simulink model "split_junction_test"  (R2014b)
settings: Solver=ode23tb  StartTime=0.0  StopTime=200  RelTol=1e-3
libraries: DAEMOT_Lib x8
settings Model: Creator=pangbor2  LastModifiedBy=koeln2

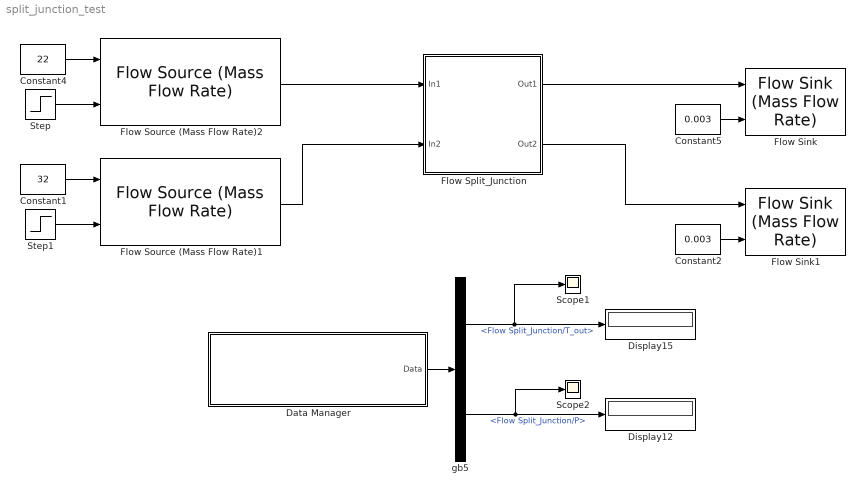
== system split_junction_test ==
  Constant1 : Constant  Value=32
  Constant2 : Constant  Value=0.003
  Constant4 : Constant  Value=22
  Constant5 : Constant  Value=0.003
  Data Manager : Subsystem  AncestorBlock=DAEMOT_Lib/Support Functions/Data Manager  mask{null=0}
      mask init:
      | set_param(gcb, 'LinkStatus', 'inactive')    % disable the library link
      settings: OpenFcn=data_manager
      mask Display: str ='Flow Split_Junction/T_out\nFlow Split_Junction/P'; fprintf(str)
  Display12 : Display
  Display15 : Display
  Flow Sink : DAEMOT_Lib/Components/Flow Sink (Mass Flow Rate)  M_ext=on  M=0  T_ext=on  T=0  P_ext=on  P=0
  Flow Sink1 : DAEMOT_Lib/Components/Flow Sink (Mass Flow Rate)  M_ext=on  M=0  T_ext=on  T=0  P_ext=on  P=0
  Flow Source (Mass Flow Rate)1 : DAEMOT_Lib/Components/Flow Source (Mass Flow Rate)  M_ext=on  M=0  T_ext=on  T=0  P_ext=on  P=0
  Flow Source (Mass Flow Rate)2 : DAEMOT_Lib/Components/Flow Source (Mass Flow Rate)  M_ext=on  M=0  T_ext=on  T=0  P_ext=on  P=0
  Flow Split_Junction : Subsystem  AncestorBlock=DAEMOT_Lib/Components/Flow Split_Junction  mask(Split/Junction){fld=PG50, Num_Out=2, Num_In=2, P_init=110, T_init=22, D=0.013, L=0.1, t=0.0015, E=2.4e6, v=0.4}
      mask prompts: fld "Fluid Type"; Num_Out "Number of Outlet Flows"; Num_In "Number of Inlet Flows"; P_init "Initial Pressure [kPa]"; T_init "Initial Temperature [°C]"; D "Diameter [m]"; L "Length [m]"; t "Tube Wall Thickness [m]"; E "Tube Modulus of Elasticity [kPa]"; v "Tube Poisson Ratio [-]"
      mask help: Splits and junctions flows using dynamic relationships. Note that the library link of the block is disabled when it is imported into a model.
      mask init:
      | h      = get_param(gcb,'handle');   % Get block handle
      | blk    = gcb;
      | hblock = get(h);     % Parse out handles structure
      | 
      | load('Fluids.mat');
      | Fluid = eval(['Fluid.',fld]);
      | 
      | % delete any previous inports and bus selectors
      | for i = str2num(hblock.Num_In)+1:hblock.Ports(1)
      |     delete_block([blk,'/In',num2str(i)])
      |     delete_block([blk,'/gb',num2str(i)])
      |     delete_block([blk,'/gm',num2str(i)])
      |     delete_block([blk,'/gt',num2str(i)])
      |     delete_block([blk,'/gp',num2str(i)])
      |     delete_block([blk,'/Sink',num2str(i)])
      |     delete_block([blk,'/pout',num2str(i)])
      |     delete_block([blk,'/min',num2str(i)])
      |     delete_block([blk,'/tin',num2str(i)])
      |     
      |     delete_unconnected_lines(blk)
      | end
      | 
      | % delete any previous inports and bus selectors
      | for i = str2num(hblock.Num_Out)+1:hblock.Ports(2)
      |     delete_block([blk,'/Out',num2str(i)])
      |     delete_block([blk,'/m',num2str(i)])
      |     delete_block([blk,'/t',num2str(i)])
      |     delete_block([blk,'/p',num2str(i)])
      |     delete_block([blk,'/b',num2str(i)])
      |     delete_block([blk,'/Source',num2str(i)])
      |     delete_block([blk,'/g',num2str(i)])
      |     delete_block([blk,'/mout',num2str(i)])
      |     %delete_block([blk,'/tout',num2str(i)])
      |     
      |     delete_unconnected_lines(blk)
      | end
      | 
      | set_param([blk,'/Mux_In_1'],'Inputs',hblock.Num_In)
      | set_param([blk,'/Mux_In_2'],'Inputs',hblock.Num_Out)
      | set_param([blk,'/Mux_In_3'],'Inputs',hblock.Num_In)
      | %set_param([blk,'/Mux_Out_1'],'Outputs',hblock.Num_Out)
      | 
      | % generate inports, bus selectors, and route lines to each vector concat
      | for i = hblock.Ports(1)+1:str2num(hblock.Num_In)
      |     
      |     % add blocks
      |     add_block('simulink/Ports & Subsystems/In1',   [blk,'/In',num2str(i)],    'Position',[120 i*80-25+20 150 i*80-12+20]);         % adding inport
      |     add_block([blk,'/gb1'],                        [blk,'/gb',num2str(i)],   'Position',[200 i*80-20+20-18 205 i*80-2+20+2]);         % adding inport
      |     add_block('simulink/Signal Routing/Goto',      [blk,'/gm',num2str(i)],    'Position',[260 i*80-17 340 i*80-3]);         % adding inport
      |     add_block('simulink/Signal Routing/Goto',      [blk,'/gt',num2str(i)],    'Position',[260 i*80+3 340 i*80+17]);         % adding inport
      |     add_block('simulink/Sinks/Terminator',          [blk,'/gp',num2str(i)],    'Position',[260 i*80+23 280 i*80+37]);         % adding inport
      |     add_block('DAEMOT_Lib/Support Functions/Sink',[blk,'/Sink',num2str(i)],'Position',[745 i*80-14 810 i*80+14]);         % adding inport
      |     add_block('simulink/Signal Routing/From',      [blk,'/pout',num2str(i)],    'Position',[625 i*80-14 705 i*80+14]);         % adding inport
      |     add_block('simulink/Signal Routing/From',       [blk,'/min',num2str(i)],     'Position',[935 -258+i*20 1015 -242+i*20]);         % adding inport
      |     add_block('simulink/Signal Routing/From',       [blk,'/tin',num2str(i)],     'Position',[935 1+i*20 1015 19+i*20]);         % adding inport
      |     
      |     % set goto and from tags
      |     set_param([blk,'/gm',num2str(i)],'GotoTag',char(horzcat('M_in',num2str(i))))
      |     set_param([blk,'/gt',num2str(i)],'GotoTag',char(horzcat('T_in',num2str(i))))
      |     %set_param([blk,'/gp',num2str(i)],'GotoTag',char(horzcat('P_in',num2str(i))))
      |     set_param([blk,'/pout',num2str(i)],'GotoTag',char('P'))
      |     set_param([blk,'/min',num2str(i)],'GotoTag',char(horzcat('M_in',num2str(i))))
      |     set_param([blk,'/tin',num2str(i)],'GotoTag',char(horzcat('T_in',num2str(i))))
      |     
      |     % set goto and from background colors
      |     set_param([blk,'/gm',num2str(i)],'BackgroundColor','yellow')
      |     set_param([blk,'/gt',num2str(i)],'BackgroundColor','yellow')
      |     %set_param([blk,'/gp',num2str(i)],'BackgroundColor','yellow')
      |     set_param([blk,'/min',num2str(i)],'BackgroundColor','yellow')
      |     set_param([blk,'/tin',num2str(i)],'BackgroundColor','yellow')
      |     set_param([blk,'/pout',num2str(i)],'BackgroundColor','cyan')
      |     
      |     % add lines
      |     add_line(blk,['In',num2str(i),'/1'], ['gb',num2str(i),'/1'],'AutoRouting','on')
      |     add_line(blk,['gb',num2str(i),'/1'],  ['gm',num2str(i),'/1'],'AutoRouting','on')
      |     add_line(blk,['gb',num2str(i),'/2'],  ['gt',num2str(i),'/1'],'AutoRouting','on')
      |     add_line(blk,['gb',num2str(i),'/3'],  ['gp',num2str(i),'/1'],'AutoRouting','on')
      |     add_line(blk,['pout',num2str(i),'/1'],  ['Sink',num2str(i),'/1'],'AutoRouting','on')
      |     add_line(blk,['min',num2str(i),'/1'],  ['Mux_In_1/',num2str(i)],'AutoRouting','on')
      |     add_line(blk,['tin',num2str(i),'/1'],  ['Mux_In_3/',num2str(i)],'AutoRouting','on')
      |     
      | end
      | 
      | % generate inports, bus selectors, and route lines to each vector concat
      | for i = hblock.Ports(2)+1:str2num(hblock.Num_Out)
      |     
      |     % add blocks
      |     add_block('simulink/Ports & Subsystems/Out1',   [blk,'/Out',num2str(i)],   'Position',[30 i*80-25+20 60 i*80-12+20]);         % adding inport
      |     add_block('simulink/Signal Routing/From',       [blk,'/m',num2str(i)],     'Position',[-150 i*80-20 -70 i*80-2]);         % adding inport
      |     add_block('simulink/Signal Routing/From',       [blk,'/t',num2str(i)],     'Position',[-150 i*80-20+20 -70 i*80-2+20]);         % adding inport
      |     add_block('simulink/Signal Routing/From',       [blk,'/p',num2str(i)],     'Position',[-150 i*80-20+40 -70 i*80-2+40]);         % adding inport
      |     add_block('simulink/Signal Routing/Bus Creator',[blk,'/b',num2str(i)],     'Position',[5 i*80-20+20-18 10 i*80-2+20+2]);         % adding inport
      |     add_block('DAEMOT_Lib/Support Functions/Source',[blk,'/Source',num2str(i)],'Position',[395 i*80-14 460 i*80+14]);         % adding inport
      |     add_block('simulink/Signal Routing/Goto',       [blk,'/g',num2str(i)],     'Position',[505 i*80-9 585 i*80+9]);         % adding inport
      |     add_block('simulink/Signal Routing/From',       [blk,'/mout',num2str(i)],  'Position',[935 -129+i*20 1015 -111+i*20]);         % adding inport
      |     %add_block('simulink/Signal Routing/Goto',      [blk,'/tout',num2str(i)],   'Position',[1455 -259+i*20 1535 -241+i*20]);         % adding inport
      |     
      |     % set goto and from tags
      |     set_param([blk,'/m',num2str(i)],'GotoTag',char(horzcat('M_out',num2str(i))))
      |     %set_param([blk,'/t',num2str(i)],'GotoTag',char(horzcat('T_out',num2str(i))))
      |     set_param([blk,'/t',num2str(i)],'GotoTag',char('T'))
      |     set_param([blk,'/p',num2str(i)],'GotoTag',char('P'))
      |     set_param([blk,'/g',num2str(i)],'GotoTag',char(horzcat('M_out',num2str(i))))
      |     set_param([blk,'/mout',num2str(i)],'GotoTag',char(horzcat('M_out',num2str(i))))
      |     %set_param([blk,'/tout',num2str(i)],'GotoTag',char(horzcat('T_out',num2str(i))))
      |     set_param([blk,'/b',num2str(i)],'Inputs','3')
      |     
      |     % set goto and from background colors
      |     set_param([blk,'/t',num2str(i)],'BackgroundColor','cyan')
      |     set_param([blk,'/m',num2str(i)],'BackgroundColor','cyan')
      |     set_param([blk,'/p',num2str(i)],'BackgroundColor','cyan')
      |     set_param([blk,'/g',num2str(i)],'BackgroundColor','cyan')
      |     set_param([blk,'/mout',num2str(i)],'BackgroundColor','cyan')
      |     %set_param([blk,'/tout',num2str(i)],'BackgroundColor','cyan')
      |     
      |     % add lines
      |     add_line(blk,['m',num2str(i),'/1'],['b',num2str(i),'/1'],'AutoRouting','on')
      |     p = get_param([blk,'/m',num2str(i)],'PortHandles');
      |     l = get_param(p.Outport,'Line');
      |     set_param(l,'Name','mdot_kgps')
      |     
      |     add_line(blk,['t',num2str(i),'/1'],['b',num2str(i),'/2'],'AutoRouting','on')
      |     p = get_param([blk,'/t',num2str(i)],'PortHandles');
      |     l = get_param(p.Outport,'Line');
      |     set_param(l,'Name','T_C')
      |     
      |     add_line(blk,['p',num2str(i),'/1'],['b',num2str(i),'/3'],'AutoRouting','on')
      |     p = get_param([blk,'/p',num2str(i)],'PortHandles');
      |     l = get_param(p.Outport,'Line');
      |     set_param(l,'Name','P_kPa')
      |     
      |     add_line(blk,['b',num2str(i),'/1'],['Out',num2str(i),'/1'],'AutoRouting','on')
      |     add_line(blk,['Source',num2str(i),'/1'],['g',num2str(i),'/1'],'AutoRouting','on')
      |     add_line(blk,['mout',num2str(i),'/1'],  ['Mux_In_2/',num2str(i)],'AutoRouting','on')
      |     %add_line(blk,['Mux_Out_1/',num2str(i)], ['tout',num2str(i),'/1'],'AutoRouting','on')
      | end
      | 
      | try
      |     set_param([blk,'/Selector1'],'InputPortWidth',num2str(hblock.Num_In))
      |     
      |     selector_str = '[1 ';
      |     for i = 2:str2num(hblock.Num_In)
      |         selector_str = [selector_str,num2str(i),' '];
      |     end
      |     selector_str = [selector_str,']'];
      |     set_param([blk,'/Selector1'],'IndexParamArray',{selector_str})%num2cell(1:hblock.Num_In))
      | catch
      |     selector_str = '[1 ';
      |     for i = 2:str2num(hblock.Num_In)
      |         selector_str = [selector_str,num2str(i),' '];
      |     end
      |     selector_str = [selector_str,']'];
      |     set_param([blk,'/Selector1'],'IndexParamArray',{selector_str})%num2cell(1:hblock.Num_In))
      |     
      |     set_param([blk,'/Selector1'],'InputPortWidth',num2str(hblock.Num_In))
      | end 
      |     
      |     clear h blk hblock
      settings: CopyFcn=|
      | h      = get_param(gcb,'handle');   % Get block handle
      | blk    = gcb;
      | 
      | set_param(blk, 'LinkStatus', 'inactive')
      settings: OpenFcn=|
      | load('Fluids.mat');
      | Set_Fluid_Popup_Names( Fluid )
      mask TypeOptions fld: Fuel | Water | Air | PG50
      mask DialogControl Container15 Prompt: Component Sizing - Nominal Values
      mask Display:
      | image(imread('Split.jpg'));
      | 
      | text(0.5,0.95,['{\bf',fld,' Split/Junction}'],'TexMode','on','horizontalAlignment', 'center')
      | text(0.5,0.08,['{(P)}'],'TexMode','on','horizontalAlignment', 'center')
      | 
      | h      = get_param(gcb,'handle');   % Get block handle
      | blk    = gcb;
      | hblock = get(h);     % Parse out handles structure
      | for i = 1:str2num(hblock.Num_In)
      |     port_label('input',i,horzcat('Flow In #',num2str(i)))
      | end
      | for i = 1:str2num(hblock.Num_Out)
      |     port_label('output',i,horzcat('Flow Out #',num2str(i)))
      | end
  Scope1 : Scope
  Scope2 : Scope
  Step : Step  Time=100  Before=.002  After=.003  SampleTime=0
  Step1 : Step  Time=100  Before=.004  After=.003  SampleTime=0
  gb5 : BusSelector  OutputSignals=Flow Split_Junction/T_out,Flow Split_Junction/P
  wires:
  Constant5/1 -> Flow Sink/2
  Flow Split_Junction/1(Out1) -> Flow Sink/1
  Flow Source (Mass Flow Rate)2/1 -> Flow Split_Junction/1(In1)
  Constant2/1 -> Flow Sink1/2
  Flow Split_Junction/2(Out2) -> Flow Sink1/1
  Flow Source (Mass Flow Rate)1/1 -> Flow Split_Junction/2(In2)
  Data Manager/1(Data) -> gb5/1
  gb5/2 -> Display12/1, Scope2/1  "<Flow Split_Junction/P>"
  gb5/1 -> Display15/1, Scope1/1  "<Flow Split_Junction/T_out>"
  Constant4/1 -> Flow Source (Mass Flow Rate)2/1
  Constant1/1 -> Flow Source (Mass Flow Rate)1/1
  Step/1 -> Flow Source (Mass Flow Rate)2/2
  Step1/1 -> Flow Source (Mass Flow Rate)1/2

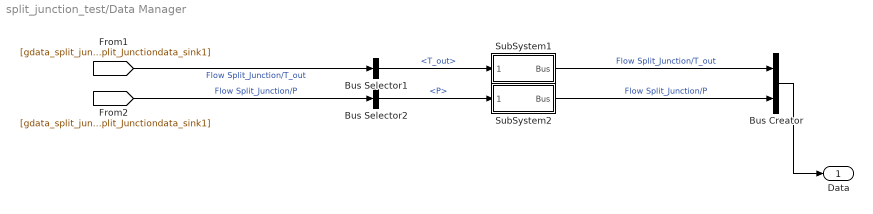
== system split_junction_test/Data Manager ==
  Bus Creator : BusCreator  Inputs=2
  Bus Selector1 : BusSelector  OutputSignals=T_out
  Bus Selector2 : BusSelector  OutputSignals=P
  SubSystem1 : Subsystem
  SubSystem2 : Subsystem
  Data : Outport
  wires:
  Bus Creator/1 -> Data/1
  [gdata_split_junction_testFlowSplit_Junctiondata_sink1] -> Bus Selector1/1  "Flow Split_Junction/T_out"
  Bus Selector1/1 -> SubSystem1/1(Rename)  "<T_out>"
  SubSystem1/1(Bus) -> Bus Creator/1  "Flow Split_Junction/T_out"
  [gdata_split_junction_testFlowSplit_Junctiondata_sink1] -> Bus Selector2/1  "Flow Split_Junction/P"
  Bus Selector2/1 -> SubSystem2/1(Rename)  "<P>"
  SubSystem2/1(Bus) -> Bus Creator/2  "Flow Split_Junction/P"

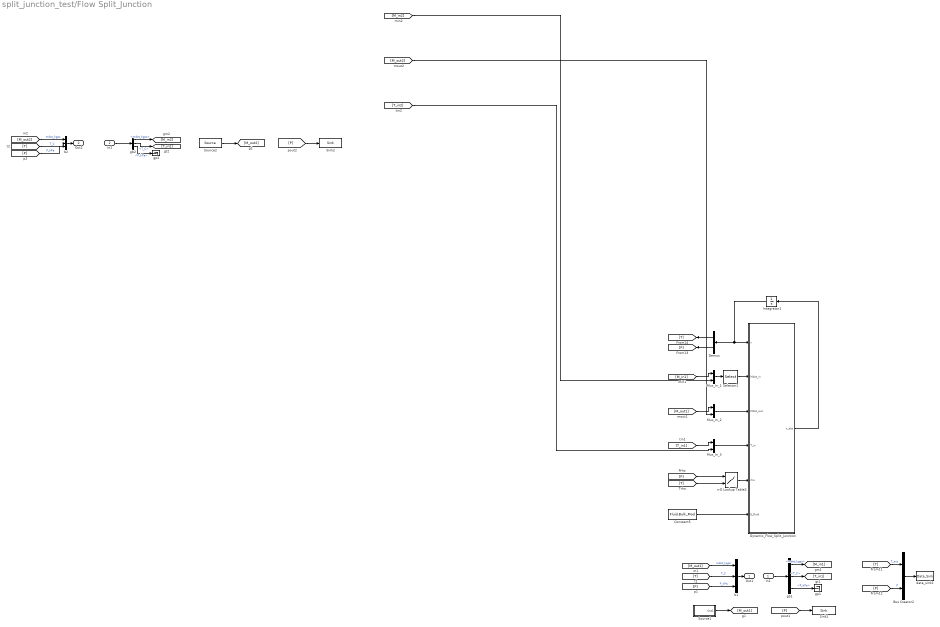
== system split_junction_test/Flow Split_Junction ==
  In1 : Inport
  In2 : Inport  Port=2
  Bus Creator2 : BusCreator  Inputs=2
  Constant5 : Constant  Value=Fluid.Bulk_Mod
  Demux : Demux  Outputs=2
  Dynamic_Flow_Split_Junction : MATLAB Function  TreatAsAtomicUnit=on
  Integrator1 : Integrator  InitialCondition=[T_init P_init]
  Mux_In_1 : Mux  Inputs=2
  Mux_In_2 : Mux  Inputs=2
  Mux_In_3 : Mux  Inputs=2
  Selector1 : Selector  InputPortWidth=2  Indices=[1 2 ]
  Sink1 : DAEMOT_Lib/Support Functions/Sink
  Sink2 : DAEMOT_Lib/Support Functions/Sink
  Source1 : Subsystem
      mask init:
      | n_src = gcb;
      | n_src = str2num(n_src(end));
      | 
      | rev_comms_source(n_src);
      mask Display: text(0.25,0.5,'Source')
  Source2 : DAEMOT_Lib/Support Functions/Source
  b1 : BusCreator  Inputs=3
  b2 : BusCreator  Inputs=3
  data_sink1 : DAEMOT_Lib/Support Functions/Data_Sink
  gb1 : BusSelector  OutputSignals=mdot_kgps,T_C,P_kPa
  gb2 : BusSelector  OutputSignals=mdot_kgps,T_C,P_kPa
  gp1 : Terminator
  gp2 : Terminator
  n-D Lookup Table2 : Lookup_n-D  BreakpointsForDimension1=Fluid.P  BreakpointsForDimension2=Fluid.T  BreakpointsForDimension3=[5, 7]  Table=Fluid.Rho_pt  ExtrapMethod=Clip  UseLastTableValue=on  RndMeth=Simplest  InputSameDT=on
  Out1 : Outport
  Out2 : Outport  Port=2
  wires:
  b1/1 -> Out1/1
  [M_out1] -> b1/1  "mdot_kgps"
  gb1/2 -> [T_in1]  "<T_C>"
  [T] -> b1/2  "T_C"
  gb1/1 -> [M_in1]  "<mdot_kgps>"
  Source1/1(Out1) -> [M_out1]
  In1/1 -> gb1/1
  [P] -> b1/3  "P_kPa"
  gb1/3 -> gp1/1  "<P_kPa>"
  Mux_In_3/1 -> Dynamic_Flow_Split_Junction/4(T_in)
  Mux_In_1/1 -> Selector1/1
  Mux_In_2/1 -> Dynamic_Flow_Split_Junction/3(Mdot_out)
  [M_in1] -> Mux_In_1/1
  [M_out1] -> Mux_In_2/1
  [T_in1] -> Mux_In_3/1
  [P] -> Sink1/1
  Dynamic_Flow_Split_Junction/1(x_dot) -> Integrator1/1
  Bus Creator2/1 -> data_sink1/1
  [T] -> Bus Creator2/1  "T_out"
  [P] -> Bus Creator2/2  "P"
  Integrator1/1 -> Demux/1, Dynamic_Flow_Split_Junction/1(x)
  Selector1/1 -> Dynamic_Flow_Split_Junction/2(Mdot_in)
  Constant5/1 -> Dynamic_Flow_Split_Junction/6(E_fluid)
  n-D Lookup Table2/1 -> Dynamic_Flow_Split_Junction/5(rho)
  [P] -> n-D Lookup Table2/1
  [T] -> n-D Lookup Table2/2
  Demux/1 -> [T]
  Demux/2 -> [P]
  In2/1 -> gb2/1
  gb2/1 -> [M_in2]  "<mdot_kgps>"
  gb2/2 -> [T_in2]  "<T_C>"
  gb2/3 -> gp2/1  "<P_kPa>"
  [P] -> Sink2/1
  [M_in2] -> Mux_In_1/2
  [T_in2] -> Mux_In_3/2
  [M_out2] -> b2/1  "mdot_kgps"
  [T] -> b2/2  "T_C"
  [P] -> b2/3  "P_kPa"
  b2/1 -> Out2/1
  Source2/1 -> [M_out2]
  [M_out2] -> Mux_In_2/2

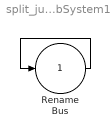
== system split_junction_test/Data Manager/SubSystem1 ==
  Rename : Inport
  Bus : Outport
  wires:
  Rename/1 -> Bus/1

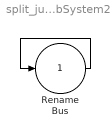
== system split_junction_test/Data Manager/SubSystem2 ==
  Rename : Inport
  Bus : Outport
  wires:
  Rename/1 -> Bus/1

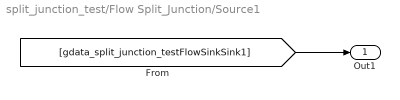
== system split_junction_test/Flow Split_Junction/Source1 ==
  Out1 : Outport
  wires:
  [gdata_split_junction_testFlowSinkSink1] -> Out1/1

== matlab function split_junction_test/Flow Split_Junction/Dynamic_Flow_Split_Junction ==
  data: x input; Mdot_in input; Mdot_out input; T_in input; x_dot output; D parameter; L parameter; t parameter; E parameter; v parameter; rho input; E_fluid input
function x_dot  = Dynamic_Flow_Split_Junction(x,Mdot_in,Mdot_out,T_in,D,L,t,E,v,rho,E_fluid)

% Constants and Conversions
Mdot_in_tot     = sum(Mdot_in);     % Total mass flow rate in
Mdot_out_tot    = sum(Mdot_out);    % Total mass flow rate out
V               = pi*D^2/4*L;       % Volume

% Parse states
T      = x(1);                  % Temperature of the tank
P      = x(2);                  % Pressure at bottom of the tank

% Calculate state derivatives
T_dot = (dot(Mdot_in,T_in)-sum(Mdot_in)*T)/(rho*V);  % Split/Junc temperature
P_dot = (Mdot_in_tot-Mdot_out_tot)/(V*rho*(1/E_fluid+D*(1-v/2)/(t*E))); % Split/Junc pressure

% Mux state derivatives
x_dot  = [T_dot,P_dot];

end
